simulink model "Stanza"  (R2025b)
settings: Solver=VariableStepAuto  StartTime=0.0  StopTime=10.0  RelTol=1e-3
values from neighbouring files (symbols this model uses):
  x_ref = op.States(1).x    [MPC.m]    (also in MPC_uguaglianza.m; calcola_N_massimo_cis.m = [289; 289; 289; 100; 100; 100]; test_K.m = [289; 289; 289; 100; 100; 100]; trova_N_controllable.m = [289; 289; 289; 100; 100; 100])
settings Model: Creator=leonardoleggeri  LastModifiedBy=leonardoleggeri

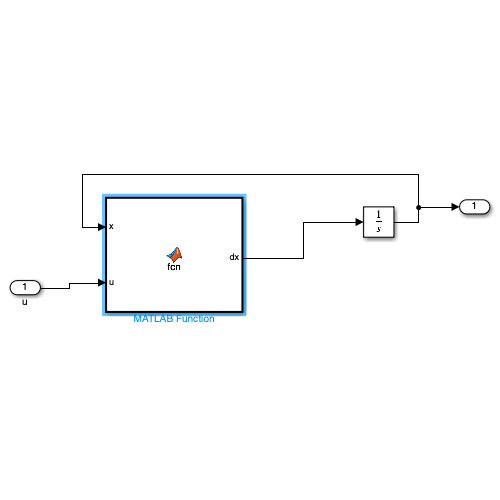
[thumbnail: Simulink's stored preview of the top-level diagram]
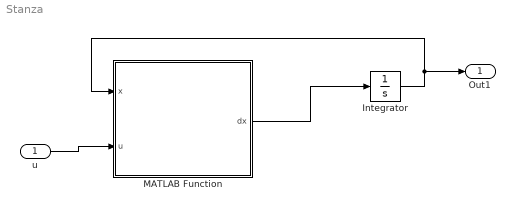
== system Stanza ==
  u : Inport  PortDimensions=3
  Integrator : Integrator  InitialCondition=x_ref
  MATLAB Function : MATLAB Function  TreatAsAtomicUnit=on
  Out1 : Outport
  wires:
  MATLAB Function/1(dx) -> Integrator/1
  Integrator/1 -> Out1/1, MATLAB Function/1(x)
  u/1 -> MATLAB Function/2(u)

== matlab function Stanza/MATLAB Function ==
  data: x input; u input; dx output
function dx = fcn(x, u)
    % Estrazione stati e ingressi
    T1 = x(1); T2 = x(2); T3 = x(3);
    Q1 = x(4); Q2 = x(5); Q3 = x(6);
    Q1_r = u(1); Q2_r = u(2); Q3_r = u(3);

    % Parametri
    C1 = 6300; C2 = 4600; C3 = 4200;
    k1_bar = 16; k2_bar = 18; k3_bar = 19;
    kext = 9; Text = 278;
    tau1 = 580; tau2 = 520; tau3 = 540;

    % Coefficienti non lineari (con abs invece della norma)
    k12 = k1_bar + 4 / (1 + exp(-0.5 * abs(T1 - T2)));
    k13 = k2_bar + 4 / (1 + exp(-0.5 * abs(T1 - T3)));
    k23 = k3_bar + 4 / (1 + exp(-0.5 * abs(T2 - T3)));

    % Equazioni differenziali (Dinamica)
    dT1 = (Q1 - k12*(T1 - T2) - k13*(T1 - T3) - kext*(T1 - Text)) / C1;
    dT2 = (Q2 + k12*(T1 - T2) - k23*(T2 - T3) - kext*(T2 - Text)) / C2;
    dT3 = (Q3 + k13*(T1 - T3) + k23*(T2 - T3) - kext*(T3 - Text)) / C3;

    dQ1 = (Q1_r - Q1) / tau1;
    dQ2 = (Q2_r - Q2) / tau2;
    dQ3 = (Q3_r - Q3) / tau3;

    dx = [dT1; dT2; dT3; dQ1; dQ2; dQ3];
end
